simulink model "SLWF_Harness"  (R2022b)
settings: configuration reference "CommonModelConfiguration" (kept outside this file)
undefined symbols (not defined in the file): cc_param_251, LCFG_ISA_Intervention_Timeout, LCFG_ISAReactivation, LCFG_ISASoundRequest, LCFG_SLWF_Deactivation_Timeout, LCFG_VehicleBrand
settings Model: Creator=AJOSHI11  LastModifiedBy=AJOSHI11
settings ConfigSetRef: SourceName=CommonModelConfiguration  SourceLocation=Base Workspace

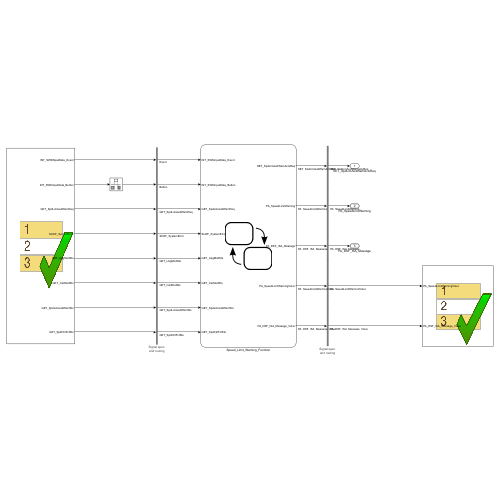
[thumbnail: Simulink's stored preview of the top-level diagram]
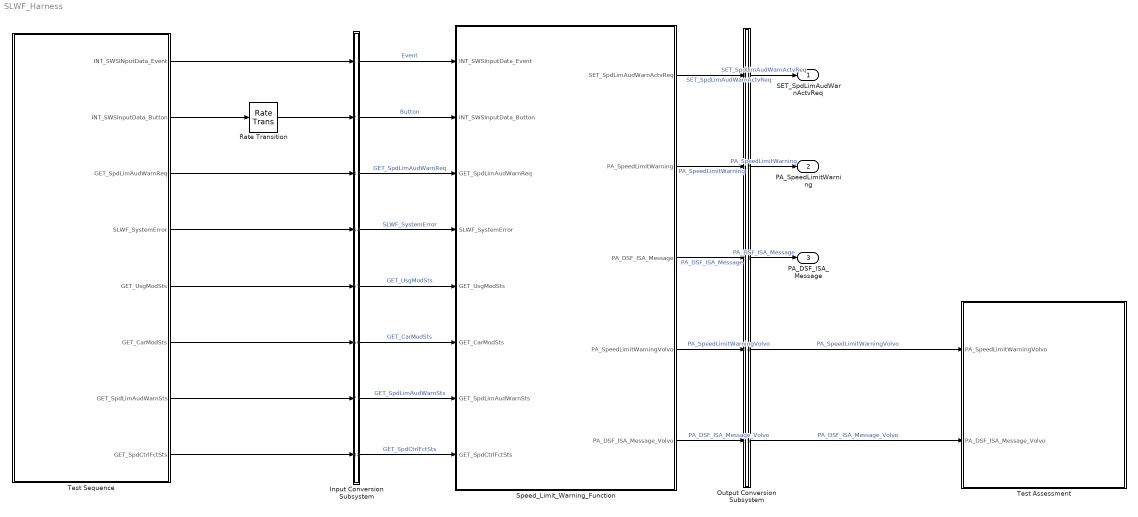
== system SLWF_Harness ==
  Input Conversion Subsystem : Subsystem  Tag=__SLT_ICS__  Description=|
      | Signal spec.
      | and routing
      settings: AttributesFormatString=%<Description>
  Output Conversion Subsystem : Subsystem  Tag=__SLT_OCS__  Description=|
      | Signal spec.
      | and routing
      settings: AttributesFormatString=%<Description>
  Rate Transition : RateTransition
  Speed_Limit_Warning_Function : Stateflow chart  TreatAsAtomicUnit=on
  Test Assessment : Test Sequence  TreatAsAtomicUnit=on
  Test Sequence : Test Sequence  TreatAsAtomicUnit=on
  SET_SpdLimAudWarnActvReq : Outport
  PA_SpeedLimitWarning : Outport  Port=2  OutDataTypeStr=Bus: PA_StatusAndWarningAndOffOnValue
  PA_DSF_ISA_Message : Outport  Port=3  OutDataTypeStr=Bus: PA_StatusAndOffOnValue
  wires:
  Output Conversion Subsystem/1(Outport_1) -> SET_SpdLimAudWarnActvReq/1  "SET_SpdLimAudWarnActvReq"
  Output Conversion Subsystem/2(Outport_2) -> PA_SpeedLimitWarning/1  "PA_SpeedLimitWarning"
  Output Conversion Subsystem/3(Outport_3) -> PA_DSF_ISA_Message/1  "PA_DSF_ISA_Message"
  Input Conversion Subsystem/1(Outport_1) -> Speed_Limit_Warning_Function/1(INT_SWSInputData_Event)  "Event"
  Input Conversion Subsystem/2(Outport_2) -> Speed_Limit_Warning_Function/2(INT_SWSInputData_Button)  "Button"
  Input Conversion Subsystem/3(Outport_3) -> Speed_Limit_Warning_Function/3(GET_SpdLimAudWarnReq)  "GET_SpdLimAudWarnReq"
  Input Conversion Subsystem/4(Outport_4) -> Speed_Limit_Warning_Function/4(SLWF_SystemError)  "SLWF_SystemError"
  Input Conversion Subsystem/5(Outport_5) -> Speed_Limit_Warning_Function/5(GET_UsgModSts)  "GET_UsgModSts"
  Input Conversion Subsystem/6(Outport_6) -> Speed_Limit_Warning_Function/6(GET_CarModSts)  "GET_CarModSts"
  Input Conversion Subsystem/7(Outport_7) -> Speed_Limit_Warning_Function/7(GET_SpdLimAudWarnSts)  "GET_SpdLimAudWarnSts"
  Input Conversion Subsystem/8(Outport_8) -> Speed_Limit_Warning_Function/8(GET_SpdCtrlFctSts)  "GET_SpdCtrlFctSts"
  Speed_Limit_Warning_Function/1(SET_SpdLimAudWarnActvReq) -> Output Conversion Subsystem/1(Inport_1)  "SET_SpdLimAudWarnActvReq"
  Speed_Limit_Warning_Function/2(PA_SpeedLimitWarning) -> Output Conversion Subsystem/2(Inport_2)  "PA_SpeedLimitWarning"
  Speed_Limit_Warning_Function/3(PA_DSF_ISA_Message) -> Output Conversion Subsystem/3(Inport_3)  "PA_DSF_ISA_Message"
  Speed_Limit_Warning_Function/4(PA_SpeedLimitWarningVolvo) -> Output Conversion Subsystem/4(Inport_4)  "PA_SpeedLimitWarningVolvo"
  Speed_Limit_Warning_Function/5(PA_DSF_ISA_Message_Volvo) -> Output Conversion Subsystem/5(Inport_5)  "PA_DSF_ISA_Message_Volvo"
  Test Sequence/1(INT_SWSINputData_Event) -> Input Conversion Subsystem/1(Inport_1)
  Test Sequence/3(GET_SpdLimAudWarnReq) -> Input Conversion Subsystem/3(Inport_3)
  Test Sequence/4(SLWF_SystemError) -> Input Conversion Subsystem/4(Inport_4)
  Test Sequence/5(GET_UsgModSts) -> Input Conversion Subsystem/5(Inport_5)
  Test Sequence/6(GET_CarModSts) -> Input Conversion Subsystem/6(Inport_6)
  Test Sequence/8(GET_SpdCtrlFctSts) -> Input Conversion Subsystem/8(Inport_8)
  Test Sequence/7(GET_SpdLimAudWarnSts) -> Input Conversion Subsystem/7(Inport_7)
  Rate Transition/1 -> Input Conversion Subsystem/2(Inport_2)
  Test Sequence/2(INT_SWSInputData_Button) -> Rate Transition/1
  Output Conversion Subsystem/4(Outport_4) -> Test Assessment/1(PA_SpeedLimitWarningVolvo)  "PA_SpeedLimitWarningVolvo"
  Output Conversion Subsystem/5(Outport_5) -> Test Assessment/2(PA_DSF_ISA_Message_Volvo)  "PA_DSF_ISA_Message_Volvo"

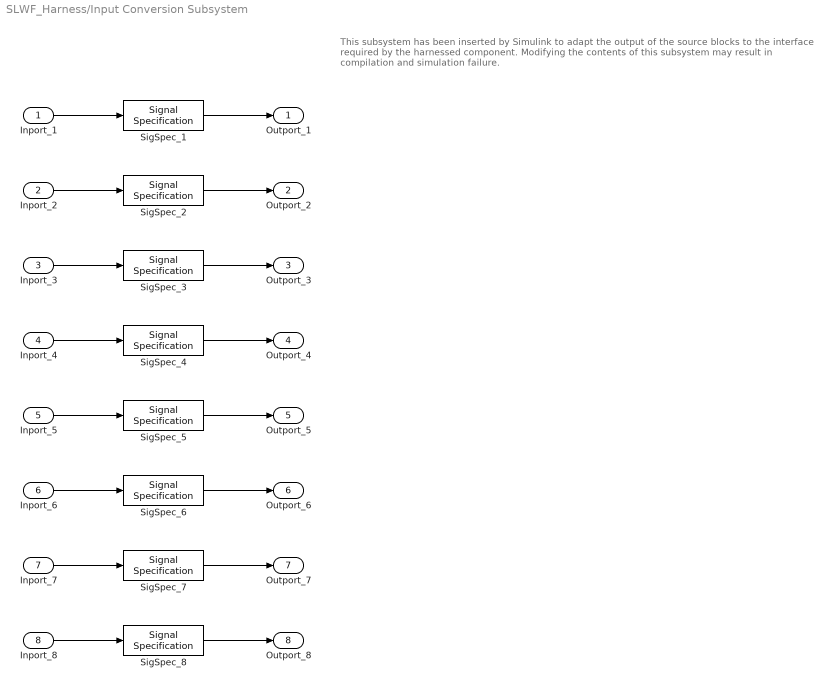
== system SLWF_Harness/Input Conversion Subsystem ==
  note: This subsystem has been inserted by Simulink to adapt the output of the source blocks to the interface required by the harnessed component.
      |  Modifying the contents of this subsystem may result in compilation and simulation failure.
  Inport_1 : Inport
  Inport_2 : Inport  Port=2
  Inport_3 : Inport  Port=3
  Inport_4 : Inport  Port=4
  Inport_5 : Inport  Port=5
  Inport_6 : Inport  Port=6
  Inport_7 : Inport  Port=7
  Inport_8 : Inport  Port=8
  SigSpec_1 : SignalSpecification  OutDataTypeStr=Enum: E_SWSEvent  Dimensions=[1]  SampleTime=[0, 0]
  SigSpec_2 : SignalSpecification  OutDataTypeStr=Enum: E_SWSButton  Dimensions=[1]  SampleTime=[0, 0]
  SigSpec_3 : SignalSpecification  OutDataTypeStr=Enum: OnOff1  Dimensions=[1]  SampleTime=[0, 0]
  SigSpec_4 : SignalSpecification  OutDataTypeStr=boolean  Dimensions=[1]  SampleTime=[0, 0]
  SigSpec_5 : SignalSpecification  OutDataTypeStr=Enum: UsgModSts1  Dimensions=[1]  SampleTime=[0, 0]
  SigSpec_6 : SignalSpecification  OutDataTypeStr=Enum: CarModSts1  Dimensions=[1]  SampleTime=[0, 0]
  SigSpec_7 : SignalSpecification  OutDataTypeStr=Enum: WarnSts  Dimensions=[1]  SampleTime=[0, 0]
  SigSpec_8 : SignalSpecification  OutDataTypeStr=Enum: FctStsSpdCtrl  Dimensions=[1]  SampleTime=[0, 0]
  Outport_1 : Outport
  Outport_2 : Outport  Port=2
  Outport_3 : Outport  Port=3
  Outport_4 : Outport  Port=4
  Outport_5 : Outport  Port=5
  Outport_6 : Outport  Port=6
  Outport_7 : Outport  Port=7
  Outport_8 : Outport  Port=8
  wires:
  SigSpec_1/1 -> Outport_1/1
  Inport_1/1 -> SigSpec_1/1
  SigSpec_2/1 -> Outport_2/1
  Inport_2/1 -> SigSpec_2/1
  SigSpec_3/1 -> Outport_3/1
  Inport_3/1 -> SigSpec_3/1
  SigSpec_4/1 -> Outport_4/1
  Inport_4/1 -> SigSpec_4/1
  SigSpec_5/1 -> Outport_5/1
  Inport_5/1 -> SigSpec_5/1
  SigSpec_6/1 -> Outport_6/1
  Inport_6/1 -> SigSpec_6/1
  SigSpec_7/1 -> Outport_7/1
  Inport_7/1 -> SigSpec_7/1
  SigSpec_8/1 -> Outport_8/1
  Inport_8/1 -> SigSpec_8/1

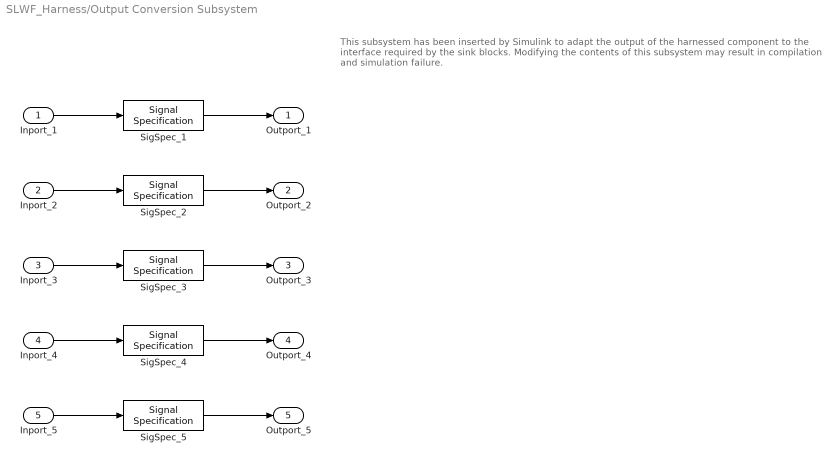
== system SLWF_Harness/Output Conversion Subsystem ==
  note: This subsystem has been inserted by Simulink to adapt the output of the harnessed component to the interface required by the sink blocks.
      |  Modifying the contents of this subsystem may result in compilation and simulation failure.
  Inport_1 : Inport
  Inport_2 : Inport  Port=2
  Inport_3 : Inport  Port=3
  Inport_4 : Inport  Port=4
  Inport_5 : Inport  Port=5
  SigSpec_1 : SignalSpecification  OutDataTypeStr=Enum: OnOff1  Dimensions=[1]
  SigSpec_2 : SignalSpecification  OutDataTypeStr=Bus: PA_StatusAndWarningAndOffOnValue  Dimensions=[1]  BusOutputAsStruct=on
  SigSpec_3 : SignalSpecification  OutDataTypeStr=Bus: PA_StatusAndOffOnValue  Dimensions=[1]  BusOutputAsStruct=on
  SigSpec_4 : SignalSpecification  OutDataTypeStr=Bus: PA_StatusAndWarningAndOffOnValue  Dimensions=[1]  BusOutputAsStruct=on
  SigSpec_5 : SignalSpecification  OutDataTypeStr=Bus: PA_StatusAndOffOnValue  Dimensions=[1]  BusOutputAsStruct=on
  Outport_1 : Outport
  Outport_2 : Outport  Port=2
  Outport_3 : Outport  Port=3
  Outport_4 : Outport  Port=4
  Outport_5 : Outport  Port=5
  wires:
  Inport_1/1 -> SigSpec_1/1
  SigSpec_1/1 -> Outport_1/1
  Inport_2/1 -> SigSpec_2/1
  SigSpec_2/1 -> Outport_2/1
  Inport_3/1 -> SigSpec_3/1
  SigSpec_3/1 -> Outport_3/1
  Inport_4/1 -> SigSpec_4/1
  SigSpec_4/1 -> Outport_4/1
  Inport_5/1 -> SigSpec_5/1
  SigSpec_5/1 -> Outport_5/1

== stateflow chart SLWF_Harness/Test Assessment ==
  state step_1
    verify(PA_DSF_ISA_Message_Volvo.Value ==E_OffOn.Off);
    verify(PA_SpeedLimitWarningVolvo.Warning==E_OffOn.Off);
    verify(PA_SpeedLimitWarningVolvo.Value==E_OffOn.Off);
    state step_1_1
    state step_1_2
    step_1 -> (junction 22) [order 1]
    (default) -> (junction 22)
    (junction 22) -> (junction 23) [order 1] : [t < 1
        | ]
    (junction 23) -> step_1_1 [order 1] : [~in(step_1.step_1_1)]
    (junction 23) -> (junction 26) [order 2]
    (junction 57) -> (junction 58)
    (junction 58) -> step_1_2 [order 1] : [~in(step_1.step_1_2)]
    (junction 58) -> (junction 61) [order 2]
    (junction 22) -> (junction 57) [order 2]
  state step_2
    verify(PA_DSF_ISA_Message_Volvo.Value==E_OffOn.Off);
    verify(PA_SpeedLimitWarningVolvo.Warning==E_OffOn.Off);
    verify(PA_SpeedLimitWarningVolvo.Value==E_OffOn.On);
    settings: description=INTERVENTION
  state step_3
    verify(PA_DSF_ISA_Message_Volvo.Value==E_OffOn.Off);
    verify(PA_SpeedLimitWarningVolvo.Warning==E_OffOn.Off);
    verify(PA_SpeedLimitWarningVolvo.Value==E_OffOn.On);
    settings: description=WAIT
  state step_4
    verify(PA_DSF_ISA_Message_Volvo.Value==E_OffOn.On);
    verify(PA_SpeedLimitWarningVolvo.Warning==E_OffOn.On);
    verify(PA_SpeedLimitWarningVolvo.Value==E_OffOn.Off);
    settings: description=MSG DISPLAY
  state step_5
    settings: description=MSG DISPLAY
    state step_5_1
      verify(PA_DSF_ISA_Message_Volvo.Value ==E_OffOn.Off);
      verify(PA_SpeedLimitWarningVolvo.Warning==E_OffOn.Off);
      verify(PA_SpeedLimitWarningVolvo.Value==E_OffOn.Off);
      settings: description=NO MSG
    state step_5_2
    (default) -> (junction 110)
    step_5 -> (junction 110) [order 1]
    (junction 110) -> (junction 111) [order 1] : [t>10
        | ]
    (junction 111) -> step_5_1 [order 1] : [~in(step_5.step_5_1)]
    (junction 111) -> (junction 114) [order 2]
    (junction 119) -> (junction 120)
    (junction 120) -> step_5_2 [order 1] : [~in(step_5.step_5_2)]
    (junction 120) -> (junction 123) [order 2]
    (junction 110) -> (junction 119) [order 2]
  state step_6
    verify(PA_DSF_ISA_Message_Volvo.Value ==E_OffOn.Off);
    verify(PA_SpeedLimitWarningVolvo.Warning==E_OffOn.Off);
    verify(PA_SpeedLimitWarningVolvo.Value==E_OffOn.On);
    settings: description=REACTIVATION
  state step_7
    settings: description=MSG DISPLAY
    state step_7_1
      verify(PA_DSF_ISA_Message_Volvo.Value==E_OffOn.On);
      verify(PA_SpeedLimitWarningVolvo.Warning==E_OffOn.On);
      verify(PA_SpeedLimitWarningVolvo.Value==E_OffOn.Off);
    state step_7_2
    (default) -> (junction 128)
    step_7 -> (junction 128) [order 1]
    (junction 128) -> (junction 129) [order 1] : [t>10
        | ]
    (junction 129) -> step_7_1 [order 1] : [~in(step_7.step_7_1)]
    (junction 129) -> (junction 132) [order 2]
    (junction 138) -> (junction 139)
    (junction 139) -> step_7_2 [order 1] : [~in(step_7.step_7_2)]
    (junction 139) -> (junction 142) [order 2]
    (junction 128) -> (junction 138) [order 2]
  state step_8
    verify(PA_DSF_ISA_Message_Volvo.Value ==E_OffOn.Off);
    verify(PA_SpeedLimitWarningVolvo.Warning==E_OffOn.Off);
    verify(PA_SpeedLimitWarningVolvo.Value==E_OffOn.Off);
    settings: description=NO MSG
  state step_9
    verify(PA_DSF_ISA_Message_Volvo.Value==E_OffOn.Off);
    verify(PA_SpeedLimitWarningVolvo.Warning==E_OffOn.Off);
    verify(PA_SpeedLimitWarningVolvo.Value==E_OffOn.On);
    settings: description=INTERVENTION
  state step_10
    verify(PA_DSF_ISA_Message_Volvo.Value==E_OffOn.Off);
    verify(PA_SpeedLimitWarningVolvo.Warning==E_OffOn.Off);
    verify(PA_SpeedLimitWarningVolvo.Value==E_OffOn.On);
    settings: description=WAIT
  state step_11
    verify(PA_DSF_ISA_Message_Volvo.Value ==E_OffOn.Off);
    verify(PA_SpeedLimitWarningVolvo.Warning==E_OffOn.Off);
    verify(PA_SpeedLimitWarningVolvo.Value==E_OffOn.Off);
    settings: description=NO MSG
  (default) -> step_1
  step_1 -> step_2 [order 1] : [
      | after(3,sec)
      | ]
  step_2 -> step_3 : [
      | after(2,sec)
      | ]
  step_3 -> step_4 : [
      | after(1,sec)
      | ]
  step_4 -> step_5 : [
      | after(1,sec)
      | ]
  step_5 -> step_6 [order 1] : [
      | after(11,sec)
      | ]
  step_6 -> step_7 : [
      | after(2,sec)
      | ]
  step_7 -> step_8 [order 1] : [
      | after(11,sec)
      | ]
  step_8 -> step_9 : [
      | after(1,sec)
      | ]
  step_9 -> step_10 : [
      | after(2,sec)
      | ]
  step_10 -> step_11 : [
      | after(3,sec)
      | ]
  data: PA_SpeedLimitWarningVolvo input; PA_DSF_ISA_Message_Volvo input

== stateflow chart SLWF_Harness/Speed_Limit_Warning_Function ==
  state CARCONFIG_INVALID
    en, du:
    SET_SpdLimAudWarnActvReq = OnOff1.OnOff1_Off;
    state CARCONFIG_INVALID_VOLVO
      en, du:
      PA_SpeedLimitWarningVolvo.Status = E_CommonStatus.NotPresent;
      PA_DSF_ISA_Message_Volvo.Status = E_CommonStatus.NotPresent;
      PA_SpeedLimitWarningVolvo.Value = E_OffOn.Off;
      PA_DSF_ISA_Message_Volvo.Value = E_OffOn.Off;
      PA_SpeedLimitWarningVolvo.Warning = E_OffOn.Off;
    state CARCONFIG_INVALID_POLESTAR
      en, du:
      PA_SpeedLimitWarning.Status = E_CommonStatus.NotPresent;
      PA_DSF_ISA_Message.Status = E_CommonStatus.NotPresent;
      PA_SpeedLimitWarning.Value = E_OffOn.Off;
      PA_DSF_ISA_Message.Value = E_OffOn.Off;
      PA_SpeedLimitWarning.Warning = E_OffOn.Off;
    (default) -> (junction 257)
    (junction 257) -> CARCONFIG_INVALID_VOLVO [order 2]
    (junction 257) -> CARCONFIG_INVALID_POLESTAR [order 1] : %Polestar
        | [LCFG_VehicleBrand == 2]
  state SYSTEM_OK
    state NOT_ACTIVE
      en, du:
      SET_SpdLimAudWarnActvReq = OnOff1.OnOff1_Off;
      state NOT_ACTIVE_VOLVO
        en, du:
        PA_SpeedLimitWarningVolvo.Status = E_CommonStatus.Disabled;
        PA_DSF_ISA_Message_Volvo.Status = E_CommonStatus.Disabled;
        PA_SpeedLimitWarningVolvo.Value = E_OffOn.Off;
        PA_DSF_ISA_Message_Volvo.Value = E_OffOn.Off;
        PA_SpeedLimitWarningVolvo.Warning = E_OffOn.Off;
      state NOT_ACTIVE_POLESTAR
        en, du:
        PA_SpeedLimitWarning.Status = E_CommonStatus.Disabled;
        PA_DSF_ISA_Message.Status = E_CommonStatus.Disabled;
        PA_SpeedLimitWarning.Value = E_OffOn.Off;
        PA_DSF_ISA_Message.Value = E_OffOn.Off;
        PA_SpeedLimitWarning.Warning = E_OffOn.Off;
      (default) -> (junction 251)
      (junction 251) -> NOT_ACTIVE_VOLVO [order 2]
      (junction 251) -> NOT_ACTIVE_POLESTAR [order 1] : %Polestar
          | [LCFG_VehicleBrand == 2]
    state ACTIVE
      state BUTTON_INTERACTION [parallel]
        settings: executionOrder=1
        state REQUEST_ON
          en, du: SET_SpdLimAudWarnActvReq = OnOff1.OnOff1_On;
        state REQUEST_OFF
          en, du: SET_SpdLimAudWarnActvReq = OnOff1.OnOff1_Off;
        (default) -> REQUEST_OFF
        REQUEST_OFF -> REQUEST_ON : %Button L2 pressed
            | [INT_SWSInputData_Button == E_SWSButton.BtnL2Req &&...
            | hasChangedTo(INT_SWSInputData_Event, E_SWSEvent.Push)]
        REQUEST_ON -> REQUEST_OFF : %Request times out
            | after(LCFG_ISASoundRequest, sec)
      state DSF_MESSAGES [parallel]
        settings: executionOrder=2
        state DSF_MESSAGE_VOLVO
          en, du:
          PA_SpeedLimitWarning.Status = E_CommonStatus.Disabled;
          PA_DSF_ISA_Message.Status = E_CommonStatus.Disabled;
          PA_SpeedLimitWarningVolvo.Status = E_CommonStatus.Available;
          PA_DSF_ISA_Message_Volvo.Status = E_CommonStatus.Available;
          state INTERVENTION
            en, du:
            PA_DSF_ISA_Message_Volvo.Value = E_OffOn.Off;
            PA_SpeedLimitWarningVolvo.Warning = E_OffOn.Off;
            PA_SpeedLimitWarningVolvo.Value = E_OffOn.On;
          state NO_MESSAGE
            en, du:
            PA_DSF_ISA_Message_Volvo.Value = E_OffOn.Off;
            PA_SpeedLimitWarningVolvo.Warning = E_OffOn.Off;
            PA_SpeedLimitWarningVolvo.Value = E_OffOn.Off;
          state MESSAGE_DISPLAYED
            en, du:
            PA_DSF_ISA_Message_Volvo.Value = E_OffOn.On;
            PA_SpeedLimitWarningVolvo.Warning = E_OffOn.On;
            PA_SpeedLimitWarningVolvo.Value = E_OffOn.Off;
          state WAIT
          state REACTIVATION_ICON
            en, du:
            PA_DSF_ISA_Message_Volvo.Value = E_OffOn.Off;
            PA_SpeedLimitWarningVolvo.Warning = E_OffOn.Off;
            PA_SpeedLimitWarningVolvo.Value = E_OffOn.On;
          (default) -> SYSTEM_OK.ACTIVE.DSF_MESSAGES.DSF_MESSAGE_VOLVO.NO_MESSAGE
          SYSTEM_OK.ACTIVE.DSF_MESSAGES.DSF_MESSAGE_VOLVO.NO_MESSAGE -> SYSTEM_OK.ACTIVE.DSF_MESSAGES.DSF_MESSAGE_VOLVO.INTERVENTION [order 3] : %Intervention from either sound or accelerator pedal response
              | [GET_SpdLimAudWarnReq == OnOff1.OnOff1_On ||...
              | GET_SpdCtrlFctSts == FctStsSpdCtrl.FctStsSpdCtrl_ActiveControlling]
          SYSTEM_OK.ACTIVE.DSF_MESSAGES.DSF_MESSAGE_VOLVO.NO_MESSAGE -> SYSTEM_OK.ACTIVE.DSF_MESSAGES.DSF_MESSAGE_VOLVO.MESSAGE_DISPLAYED [order 1] : %ISA has been turned Off
              | [hasChangedFrom(GET_SpdLimAudWarnSts, WarnSts.WarnSts_ON) &&...
              | hasChangedTo(GET_SpdLimAudWarnSts, WarnSts.WarnSts_OFF)]
          SYSTEM_OK.ACTIVE.DSF_MESSAGES.DSF_MESSAGE_VOLVO.MESSAGE_DISPLAYED -> SYSTEM_OK.ACTIVE.DSF_MESSAGES.DSF_MESSAGE_VOLVO.NO_MESSAGE [order 2] : %Timer has elapsed OR ISA has been turned On before timer has elapsed
              | [after(LCFG_SLWF_Deactivation_Timeout, sec)]
          SYSTEM_OK.ACTIVE.DSF_MESSAGES.DSF_MESSAGE_VOLVO.INTERVENTION -> SYSTEM_OK.ACTIVE.DSF_MESSAGES.DSF_MESSAGE_VOLVO.WAIT [order 2] : %Intervention stopped but shown at least LCFG time before removing it in display
              | [GET_SpdLimAudWarnReq == OnOff1.OnOff1_Off &&...
              | GET_SpdCtrlFctSts ~= FctStsSpdCtrl.FctStsSpdCtrl_ActiveControlling]
          SYSTEM_OK.ACTIVE.DSF_MESSAGES.DSF_MESSAGE_VOLVO.WAIT -> SYSTEM_OK.ACTIVE.DSF_MESSAGES.DSF_MESSAGE_VOLVO.NO_MESSAGE [order 2] : [after(LCFG_ISA_Intervention_Timeout, sec)]
          SYSTEM_OK.ACTIVE.DSF_MESSAGES.DSF_MESSAGE_VOLVO.WAIT -> (junction 267) [order 1] : [%ISA has been turned Off
              | [hasChangedFrom(GET_SpdLimAudWarnSts, WarnSts.WarnSts_ON) &&...
              | hasChangedTo(GET_SpdLimAudWarnSts, WarnSts.WarnSts_OFF)]]
          SYSTEM_OK.ACTIVE.DSF_MESSAGES.DSF_MESSAGE_VOLVO.NO_MESSAGE -> SYSTEM_OK.ACTIVE.DSF_MESSAGES.DSF_MESSAGE_VOLVO.REACTIVATION_ICON [order 2] : %ISA turned on again, reactivation icon(on) displayed
              | [hasChangedFrom(GET_SpdLimAudWarnSts, WarnSts.WarnSts_OFF) &&...
              | hasChangedTo(GET_SpdLimAudWarnSts, WarnSts.WarnSts_ON)]
          SYSTEM_OK.ACTIVE.DSF_MESSAGES.DSF_MESSAGE_VOLVO.REACTIVATION_ICON -> SYSTEM_OK.ACTIVE.DSF_MESSAGES.DSF_MESSAGE_VOLVO.NO_MESSAGE [order 2] : %Reactivation icon timing out after LCFG seconds
              | [after(LCFG_ISAReactivation, sec)]
          SYSTEM_OK.ACTIVE.DSF_MESSAGES.DSF_MESSAGE_VOLVO.INTERVENTION -> (junction 267) [order 1] : [%ISA has been turned Off
              | [hasChangedFrom(GET_SpdLimAudWarnSts, WarnSts.WarnSts_ON) &&...
              | hasChangedTo(GET_SpdLimAudWarnSts, WarnSts.WarnSts_OFF)]]
          SYSTEM_OK.ACTIVE.DSF_MESSAGES.DSF_MESSAGE_VOLVO.MESSAGE_DISPLAYED -> SYSTEM_OK.ACTIVE.DSF_MESSAGES.DSF_MESSAGE_VOLVO.REACTIVATION_ICON [order 1] : %ISA turned on again, reactivation icon(on) displayed
              | [hasChangedFrom(GET_SpdLimAudWarnSts, WarnSts.WarnSts_OFF) &&...
              | hasChangedTo(GET_SpdLimAudWarnSts, WarnSts.WarnSts_ON)]
          SYSTEM_OK.ACTIVE.DSF_MESSAGES.DSF_MESSAGE_VOLVO.REACTIVATION_ICON -> SYSTEM_OK.ACTIVE.DSF_MESSAGES.DSF_MESSAGE_VOLVO.MESSAGE_DISPLAYED [order 1] : %ISA has been turned Off
              | [hasChangedFrom(GET_SpdLimAudWarnSts, WarnSts.WarnSts_ON) &&...
              | hasChangedTo(GET_SpdLimAudWarnSts, WarnSts.WarnSts_OFF)]
          (junction 267) -> SYSTEM_OK.ACTIVE.DSF_MESSAGES.DSF_MESSAGE_VOLVO.MESSAGE_DISPLAYED
        state DSF_MESSAGE_POLESTAR
          en, du:
          PA_SpeedLimitWarning.Status = E_CommonStatus.Available;
          PA_DSF_ISA_Message.Status = E_CommonStatus.Available;
          PA_SpeedLimitWarningVolvo.Status = E_CommonStatus.Disabled;
          PA_DSF_ISA_Message_Volvo.Status = E_CommonStatus.Disabled;
          state INTERVENTION
            en, du:
            PA_DSF_ISA_Message.Value = E_OffOn.Off;
            PA_SpeedLimitWarning.Warning = E_OffOn.Off;
            PA_SpeedLimitWarning.Value = E_OffOn.On;
          state NO_MESSAGE
            en, du:
            PA_DSF_ISA_Message.Value = E_OffOn.Off;
            PA_SpeedLimitWarning.Warning = E_OffOn.Off;
            PA_SpeedLimitWarning.Value = E_OffOn.Off;
          state MESSAGE_DISPLAYED
            en, du:
            PA_DSF_ISA_Message.Value = E_OffOn.On;
            PA_SpeedLimitWarning.Warning = E_OffOn.On;
            PA_SpeedLimitWarning.Value = E_OffOn.Off;
          state WAIT
          state REACTIVATION_ICON
            en, du:
            PA_DSF_ISA_Message.Value = E_OffOn.Off;
            PA_SpeedLimitWarning.Warning = E_OffOn.Off;
            PA_SpeedLimitWarning.Value = E_OffOn.On;
          (default) -> SYSTEM_OK.ACTIVE.DSF_MESSAGES.DSF_MESSAGE_POLESTAR.NO_MESSAGE
          SYSTEM_OK.ACTIVE.DSF_MESSAGES.DSF_MESSAGE_POLESTAR.NO_MESSAGE -> SYSTEM_OK.ACTIVE.DSF_MESSAGES.DSF_MESSAGE_POLESTAR.INTERVENTION [order 3] : %Intervention by sound
              | [GET_SpdLimAudWarnReq == OnOff1.OnOff1_On]
          SYSTEM_OK.ACTIVE.DSF_MESSAGES.DSF_MESSAGE_POLESTAR.MESSAGE_DISPLAYED -> SYSTEM_OK.ACTIVE.DSF_MESSAGES.DSF_MESSAGE_POLESTAR.NO_MESSAGE [order 2] : %Timer has elapsed, message and icon removed
              | [after(LCFG_SLWF_Deactivation_Timeout, sec)]
          SYSTEM_OK.ACTIVE.DSF_MESSAGES.DSF_MESSAGE_POLESTAR.NO_MESSAGE -> SYSTEM_OK.ACTIVE.DSF_MESSAGES.DSF_MESSAGE_POLESTAR.MESSAGE_DISPLAYED [order 1] : %ISA has been turned Off
              | [hasChangedFrom(GET_SpdLimAudWarnSts, WarnSts.WarnSts_ON) &&...
              | hasChangedTo(GET_SpdLimAudWarnSts, WarnSts.WarnSts_OFF)]
          SYSTEM_OK.ACTIVE.DSF_MESSAGES.DSF_MESSAGE_POLESTAR.WAIT -> SYSTEM_OK.ACTIVE.DSF_MESSAGES.DSF_MESSAGE_POLESTAR.NO_MESSAGE [order 2] : [after(LCFG_ISA_Intervention_Timeout, sec)]
          SYSTEM_OK.ACTIVE.DSF_MESSAGES.DSF_MESSAGE_POLESTAR.INTERVENTION -> SYSTEM_OK.ACTIVE.DSF_MESSAGES.DSF_MESSAGE_POLESTAR.WAIT [order 2] : %Intervention stopped but shown at least LCFG time before removing it in display
              | [GET_SpdLimAudWarnReq == OnOff1.OnOff1_Off]
          SYSTEM_OK.ACTIVE.DSF_MESSAGES.DSF_MESSAGE_POLESTAR.WAIT -> (junction 273) [order 1] : [%ISA turned Off
              | [hasChangedFrom(GET_SpdLimAudWarnSts, WarnSts.WarnSts_ON) &&...
              | hasChangedTo(GET_SpdLimAudWarnSts, WarnSts.WarnSts_OFF)]]
          SYSTEM_OK.ACTIVE.DSF_MESSAGES.DSF_MESSAGE_POLESTAR.NO_MESSAGE -> SYSTEM_OK.ACTIVE.DSF_MESSAGES.DSF_MESSAGE_POLESTAR.REACTIVATION_ICON [order 2] : %ISA turned on again, reactivation (on) icon displayed
              | [hasChangedFrom(GET_SpdLimAudWarnSts, WarnSts.WarnSts_OFF) &&...
              | hasChangedTo(GET_SpdLimAudWarnSts, WarnSts.WarnSts_ON)]
          SYSTEM_OK.ACTIVE.DSF_MESSAGES.DSF_MESSAGE_POLESTAR.REACTIVATION_ICON -> SYSTEM_OK.ACTIVE.DSF_MESSAGES.DSF_MESSAGE_POLESTAR.NO_MESSAGE [order 2] : %Reactivation icon timing out after LCFG seconds
              | [after(LCFG_ISAReactivation, sec)]
          SYSTEM_OK.ACTIVE.DSF_MESSAGES.DSF_MESSAGE_POLESTAR.INTERVENTION -> (junction 273) [order 1] : [%ISA turned Off
              | [hasChangedFrom(GET_SpdLimAudWarnSts, WarnSts.WarnSts_ON) &&...
              | hasChangedTo(GET_SpdLimAudWarnSts, WarnSts.WarnSts_OFF)]]
          SYSTEM_OK.ACTIVE.DSF_MESSAGES.DSF_MESSAGE_POLESTAR.MESSAGE_DISPLAYED -> SYSTEM_OK.ACTIVE.DSF_MESSAGES.DSF_MESSAGE_POLESTAR.REACTIVATION_ICON [order 1] : %ISA turned on again, reactivation icon (on) displayed
              | [hasChangedFrom(GET_SpdLimAudWarnSts, WarnSts.WarnSts_OFF) &&...
              | hasChangedTo(GET_SpdLimAudWarnSts, WarnSts.WarnSts_ON)]
          SYSTEM_OK.ACTIVE.DSF_MESSAGES.DSF_MESSAGE_POLESTAR.REACTIVATION_ICON -> SYSTEM_OK.ACTIVE.DSF_MESSAGES.DSF_MESSAGE_POLESTAR.MESSAGE_DISPLAYED [order 1] : %ISA has been turned off
              | [hasChangedFrom(GET_SpdLimAudWarnSts, WarnSts.WarnSts_ON) &&...
              | hasChangedTo(GET_SpdLimAudWarnSts, WarnSts.WarnSts_OFF)]
          (junction 273) -> SYSTEM_OK.ACTIVE.DSF_MESSAGES.DSF_MESSAGE_POLESTAR.MESSAGE_DISPLAYED
        (default) -> (junction 164)
        (junction 164) -> DSF_MESSAGE_VOLVO [order 2]
        (junction 164) -> DSF_MESSAGE_POLESTAR [order 1] : %Polestar
            | [LCFG_VehicleBrand == 2]
    state isActive = activationCheck [function]
      (default) -> (junction 42)
      (junction 42) -> (junction 46) [order 1] : [GET_UsgModSts == UsgModSts1.UsgModSts1_UsgModDrvg &&...
          | GET_CarModSts == CarModSts1.CarModSts1_CarModNorm]
      (junction 42) -> (junction 47) [order 2] : {isActive = false;}
      (junction 46) -> (junction 48) : {isActive = true;}
      (junction 48) -> (junction 47)
      (junction 47) -> (junction 49)
    (default) -> (junction 30)
    (junction 30) -> NOT_ACTIVE [order 1] : [~activationCheck()]
    (junction 30) -> (junction 33) [order 2]
    NOT_ACTIVE -> ACTIVE : [activationCheck()]
    ACTIVE -> NOT_ACTIVE : [~activationCheck()]
    (junction 33) -> ACTIVE
  state SYSTEM_ERROR
    en, du:
    SET_SpdLimAudWarnActvReq = OnOff1.OnOff1_Off;
    state SYSTEM_ERROR_VOLVO
      en, du:
      PA_SpeedLimitWarningVolvo.Status = E_CommonStatus.SystemError;
      PA_DSF_ISA_Message_Volvo.Status = E_CommonStatus.SystemError;
      PA_SpeedLimitWarningVolvo.Value = E_OffOn.Off;
      PA_DSF_ISA_Message_Volvo.Value = E_OffOn.Off;
      PA_SpeedLimitWarningVolvo.Warning = E_OffOn.Off;
    state SYSTEM_ERROR_POLESTAR
      en, du:
      PA_SpeedLimitWarning.Status = E_CommonStatus.SystemError;
      PA_DSF_ISA_Message.Status = E_CommonStatus.SystemError;
      PA_SpeedLimitWarning.Value = E_OffOn.Off;
      PA_DSF_ISA_Message.Value = E_OffOn.Off;
      PA_SpeedLimitWarning.Warning = E_OffOn.Off;
    (default) -> (junction 245)
    (junction 245) -> SYSTEM_ERROR_POLESTAR [order 1] : %Polestar
        | [LCFG_VehicleBrand == 2]
    (junction 245) -> SYSTEM_ERROR_VOLVO [order 2]
  (default) -> (junction 14)
  (junction 14) -> CARCONFIG_INVALID [order 2]
  (junction 14) -> (junction 17) [order 1] : [(cc_param_251 == 2||...
      | cc_param_251 == 3)]
  (junction 17) -> SYSTEM_OK [order 1] : [SLWF_SystemError == false]
  (junction 17) -> (junction 20) [order 2]
  SYSTEM_OK -> SYSTEM_ERROR : [SLWF_SystemError == true]
  SYSTEM_ERROR -> SYSTEM_OK : [SLWF_SystemError == false]
  (junction 20) -> SYSTEM_ERROR
  data: isActive function_output; INT_SWSInputData_Event input Enum: E_SWSEvent; INT_SWSInputData_Button input Enum: E_SWSButton; SET_SpdLimAudWarnActvReq output Enum: OnOff1; PA_SpeedLimitWarning output Bus: PA_StatusAndWarningAndOffOnValue; cc_param_251 parameter uint8; GET_SpdLimAudWarnReq input Enum: OnOff1; SLWF_SystemError input boolean; GET_UsgModSts input Enum: UsgModSts1; GET_CarModSts input Enum: CarModSts1; LCFG_ISASoundRequest parameter single; GET_SpdLimAudWarnSts input Enum: WarnSts; PA_DSF_ISA_Message output Bus: PA_StatusAndOffOnValue; LCFG_SLWF_Deactivation_Timeout parameter single; GET_SpdCtrlFctSts input Enum: FctStsSpdCtrl; LCFG_VehicleBrand parameter single; PA_SpeedLimitWarningVolvo output Bus: PA_StatusAndWarningAndOffOnValue; PA_DSF_ISA_Message_Volvo output Bus: PA_StatusAndOffOnValue; LCFG_ISAReactivation parameter single; LCFG_ISA_Intervention_Timeout parameter single

== stateflow chart SLWF_Harness/Test Sequence ==
  state step_1
    INT_SWSINputData_Event = E_SWSEvent.Idle;
    INT_SWSInputData_Button = E_SWSButton.None;
    GET_SpdLimAudWarnReq = OnOff1.OnOff1_Off;
    SLWF_SystemError = false;
    GET_UsgModSts = UsgModSts1.UsgModSts1_UsgModDrvg;
    GET_CarModSts = CarModSts1.CarModSts1_CarModNorm;
    GET_SpdLimAudWarnSts = WarnSts.WarnSts_ON;
    GET_SpdCtrlFctSts = FctStsSpdCtrl.FctStsSpdCtrl_Off;
    settings: description=in NO MESSAGE state
  state step_2
    INT_SWSInputData_Button = E_SWSButton.BtnL2Req;
    INT_SWSINputData_Event = E_SWSEvent.Push;
    settings: description=in NO MESSAGE state
  state step_3
    GET_SpdLimAudWarnReq = OnOff1.OnOff1_On;
    settings: description=In INTERVENTION state
  state step_4
    GET_SpdLimAudWarnReq = OnOff1.OnOff1_Off;
    settings: description=IN WAIT state
  state step_5
    INT_SWSInputData_Button = E_SWSButton.BtnL2Req;
    INT_SWSINputData_Event = E_SWSEvent.Push;
    % Triggers SpdLimAudWarnActReq whicj toggles GET_SpdLimAudWarnSts
    GET_SpdLimAudWarnSts = WarnSts.WarnSts_OFF;
    settings: description=IN MESSAGE DISPLAYED state
  state Step_6
    settings: description=In NO MESSAGE state
  state step_7
    GET_SpdLimAudWarnReq = OnOff1.OnOff1_Off;
    GET_SpdLimAudWarnSts = WarnSts.WarnSts_ON;
    settings: description=IN REACTIVATION state
  state step_8_WAIT
    GET_SpdLimAudWarnSts = WarnSts.WarnSts_OFF;
    settings: description=In MESSAGE_DSIPLAYED state
  state step_9
    settings: description=In NO_MESSAGE state
  state step_10
    GET_SpdLimAudWarnReq = OnOff1.OnOff1_On;
    settings: description=IN INTERVENTION state
  state step_11
    GET_SpdLimAudWarnReq = OnOff1.OnOff1_Off;
    settings: description=IN WAIT state
  state step_12
    settings: description=In NO MESSAGE state
  (default) -> step_1
  step_1 -> step_2 : [
      | after(2,sec)
      | ]
  step_2 -> step_3 : [
      | after(1,sec)
      | ]
  step_3 -> step_4 : [
      | after(2,sec)
      | ]
  step_4 -> step_5 : [
      | after(1,sec)
      | ]
  step_5 -> Step_6 : [
      | after(1,sec)
      | ]
  Step_6 -> step_7 : [
      | after(11,sec)
      | ]
  step_7 -> step_8_WAIT : [
      | after(2,sec)
      | ]
  step_8_WAIT -> step_9 : [
      | after(11,sec)
      | ]
  step_9 -> step_10 : [
      | after(1,sec)
      | ]
  step_10 -> step_11 : [
      | after(2,sec)
      | ]
  step_11 -> step_12 : [
      | after(3,sec)
      | ]
  data: INT_SWSINputData_Event output; INT_SWSInputData_Button output; GET_SpdLimAudWarnReq output; SLWF_SystemError output; GET_UsgModSts output; GET_CarModSts output; GET_SpdLimAudWarnSts output; GET_SpdCtrlFctSts output
